simulink model "PCM_WithoutRamp"  (R2024a)
settings: Solver=VariableStepAuto  StartTime=0.0  StopTime=.06  FixedStep=.00001  MaxStep=.000001  RelTol=1e-3
values from neighbouring files (symbols this model uses):
  C = 10*10^-6    (= 1e-05)    [parameters.m]
  Fs = 100*10^3    (= 100000)    [parameters.m]
  L = 220*10^-6    (= 0.00022)    [parameters.m]
  R = 5    [parameters.m]
libraries: simulink_extras x1, spsStairGeneratorLib x1
settings Model: Creator=User  LastModifiedBy=User
settings SolverCC: MaxConsecutiveZCs=5000
settings DebuggingCC: IgnoredZcDiagnostic=none  UnconnectedInputMsg=warning  UnconnectedOutputMsg=warning  UnconnectedLineMsg=warning
settings ModelReferenceCC: EnableRefExpFcnMdlSchedulingChecks=on
settings RTWCC: GPUComputeCapability=3.5  DLArmComputeVersion=19.05

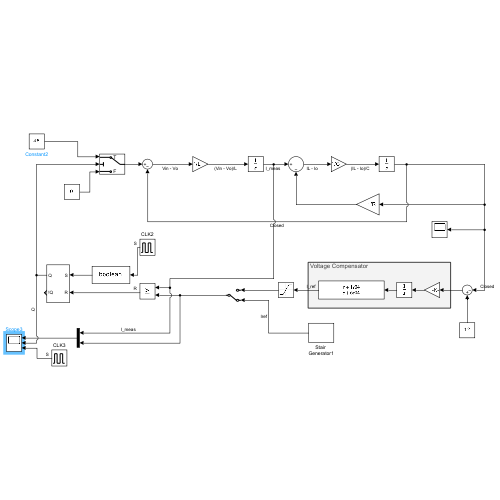
[thumbnail: Simulink's stored preview of the top-level diagram]
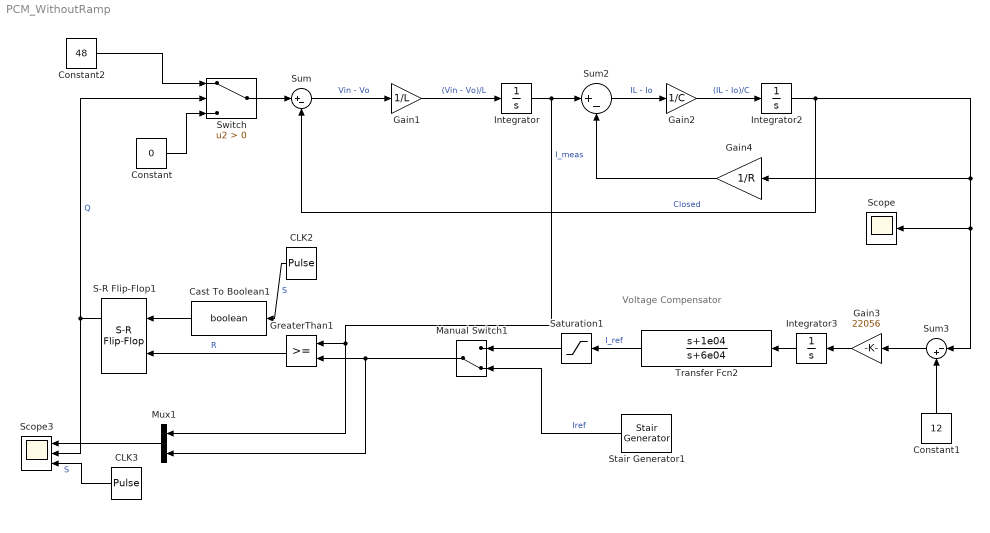
== system PCM_WithoutRamp ==
  note: Voltage Compensator
  CLK2 : DiscretePulseGenerator  PulseType=Time based  Period=1/Fs  PulseWidth=10
  CLK3 : DiscretePulseGenerator  PulseType=Time based  Period=1/Fs  PulseWidth=10
  Cast To Boolean1 : DataTypeConversion  OutDataTypeStr=boolean  SaturateOnIntegerOverflow=off  RndMeth=Floor
  Constant : Constant  Value=0
  Constant1 : Constant  Value=12
  Constant2 : Constant  Value=48
  Gain1 : Gain  Gain=1/L
  Gain2 : Gain  Gain=1/C
  Gain3 : Gain  Gain=22056
  Gain4 : Gain  Gain=1/R
  GreaterThan1 : RelationalOperator  OutDataTypeStr=boolean  RndMeth=Simplest  InputSameDT=off
  Integrator : Integrator
  Integrator2 : Integrator
  Integrator3 : Integrator
  Manual Switch1 : ManualSwitch  CurrentSetting=0
  Mux1 : Mux  Inputs=2
  S-R Flip-Flop1 : simulink_extras/Flip Flops/S-R Flip-Flop  initial_condition=0
  Saturation1 : Saturate  UpperLimit=inf  LowerLimit=0
  Scope : Scope
  Scope3 : Scope  NumInputPorts=3
  Stair Generator1 : spsStairGeneratorLib/Stair Generator  t=[0,0.03]  e=[3,6]  Ts=0
  Sum : Sum  Inputs=|+-
  Sum2 : Sum  Inputs=|+-
  Sum3 : Sum  Inputs=|-+
  Switch : Switch  Criteria=u2 > Threshold  SaturateOnIntegerOverflow=off  InputSameDT=off
  Transfer Fcn2 : TransferFcn  Numerator=[1 1e04]  Denominator=[1 6e04]
  wires:
  Sum/1 -> Gain1/1  "Vin - Vo"
  Gain4/1 -> Sum2/2
  Gain1/1 -> Integrator/1  "(Vin - Vo)/L"
  Constant/1 -> Switch/3
  Sum2/1 -> Gain2/1  "IL - Io"
  Gain2/1 -> Integrator2/1  "(IL - Io)/C"
  Constant2/1 -> Switch/1
  Switch/1 -> Sum/1
  Integrator3/1 -> Transfer Fcn2/1
  Sum3/1 -> Gain3/1
  Gain3/1 -> Integrator3/1
  Stair Generator1/1 -> Manual Switch1/2  "Iref"
  Manual Switch1/1 -> GreaterThan1/2, Mux1/2
  Integrator2/1 -> Scope/1, Sum3/1, Gain4/1, Sum/2  "Closed"
  CLK3/1 -> Scope3/3  "S"
  CLK2/1 -> Cast To Boolean1/1  "S"
  Constant1/1 -> Sum3/2
  Integrator/1 -> Sum2/1, Mux1/1, GreaterThan1/1  "I_meas"
  GreaterThan1/1 -> S-R Flip-Flop1/2  "R"
  Transfer Fcn2/1 -> Saturation1/1  "I_ref"
  Cast To Boolean1/1 -> S-R Flip-Flop1/1
  Mux1/1 -> Scope3/1
  S-R Flip-Flop1/1 -> Switch/2, Scope3/2  "Q"
  Saturation1/1 -> Manual Switch1/1
